simulink model "simulated_physical_reactor_v4_isolated"  (R2023a)
settings: Solver=FixedStepAuto  StartTime=0.0  StopTime=500  FixedStep=ts  RelTol=1e-3
values from neighbouring files (symbols this model uses):
  actionDelay = 10    [MainCode.m]
  buffer = 10    [MainCode.m]
  C0_attack_c = 0    [MainCode.m]
  C0_noise = 1    [MainCode.m]
  C0_post_attack = 0    [MainCode.m]
  C0_post_attack_val = -.25    (= -0.25)    [MainCode.m]
  Ccell0 = cell0 / v_cell    (= 15384.6153846)    [MainCode.m]
  CG0 = 185    [MainCode.m]
  CG_attack_c = 55    [MainCode.m]
  CG_attack_time = 175    [MainCode.m]
  CG_fake_failure = 0    [MainCode.m]
  CG_fake_failure_noise = 8    [MainCode.m]
  CG_increase_b = 0    [MainCode.m]
  CG_increase_rate = 2    [MainCode.m]
  cg_noGrowth = 10    [MainCode.m]
  CG_noise = 1    [MainCode.m]
  CG_post_attack = 1    [MainCode.m]
  CG_post_attack_val = .25    (= 0.25)    [MainCode.m]
  CG_ramp_attack = 1    [MainCode.m]
  CG_ramp_time = 125    [MainCode.m]
  CG_target = 50    [MainCode.m]
  CM = 4    [MainCode.m]
  CO0 = .245    (= 0.245)    [MainCode.m]
  CO_attack_time = 80    [MainCode.m]
  CO_fake_failure = 0    [MainCode.m]
  CO_fake_failure_mean = .08    (= 0.08)    [MainCode.m]
  CO_fake_failure_noise = .005    (= 0.005)    [MainCode.m]
  CO_ramp_attack = 0    [MainCode.m]
  CO_ramp_time = 100    [MainCode.m]
  count_thresh = 3    [MainCode.m]
  F_fresh_max = 25    [MainCode.m]
  F_net = F_fresh_start + F_recycle_start    (= 334.8)    [MainCode.m]
  flowrateNoiseActive = 0    [MainCode.m]
  flowrateNoiseVal = 0.5 / 100    (= 0.005)    [MainCode.m]
  fresh_attack = 0    [MainCode.m]
  fresh_attack_time = 70    [MainCode.m]
  fresh_attack_val = .1    (= 0.1)    [MainCode.m]
  freshPump_fail_time = 30    [MainCode.m]
  freshPump_failure = 0    [MainCode.m]
  freshPump_response_increases = 2    [MainCode.m]
  freshPump_response_window = 10    [MainCode.m]
  g_failure_start_t = 80    [MainCode.m]
  g_fault_wait_time = 10    [MainCode.m]
  g_flowrate_control_windowsize = 10    [MainCode.m]
  g_lownoise_val = 1.25    [MainCode.m]
  g_numpoints_fail = g_standdev_window_size+1    (= 16)    [MainCode.m]
  g_numpoints_low = 4    [MainCode.m]
  g_prob_arraylen = 15    [MainCode.m]
  g_prob_count = 6    [MainCode.m]
  g_prob_thresh = .45    (= 0.45)    [MainCode.m]
  g_standdev_window_size = 15    [MainCode.m]
  g_standev_tol = 7    [MainCode.m]
  glucose_fail_noise = 10    [MainCode.m]
  glucosesensor_failure = 0    [MainCode.m]
  lowConc_controller_onState = 1    [MainCode.m]
  mean_noise_C0 = 0    [MainCode.m]
  mean_noise_CG = 0    [MainCode.m]
  mu_max = 0.0251    [MainCode.m]
  n_size = t_window/ts    (= 2.5)    [MainCode.m]
  n_size_CG = n_size    (= 2.5)    [MainCode.m]
  o2_alpha = .20    (= 0.2)    [MainCode.m]
  o2_fail_mean = .008    (= 0.008)    [MainCode.m]
  o2_fail_noise = .005    (= 0.005)    [MainCode.m]
  o2_fail_time = 50    [MainCode.m]
  o2_fault_halfrange = .01    (= 0.01)    [MainCode.m]
  o2_fault_numpoints = 5    [MainCode.m]
  o2_lownoise_val = .0008    (= 0.0008)    [MainCode.m]
  o2_movingaverage_window = 10    [MainCode.m]
  o2_numpoints_low = 6    [MainCode.m]
  o2_prob_arraylen = 10    [MainCode.m]
  o2_prob_count = 6    [MainCode.m]
  o2_prob_thresh = .45    (= 0.45)    [MainCode.m]
  o2sensor_failure = 0    [MainCode.m]
  OCR = 2.8e-11    [MainCode.m]
  p_thresh = .4    (= 0.4)    [MainCode.m]
  rec_attack = 0    [MainCode.m]
  rec_attack_time = 50    [MainCode.m]
  rec_attack_val = 120    [MainCode.m]
  recPump_drop_val = .02    (= 0.02)    [MainCode.m]
  recPump_fail_time = 30    [MainCode.m]
  recPump_failure = 0    [MainCode.m]
  recPump_rollingavg_samples_buildup = 10    [MainCode.m]
  recPump_smallDrop_size = 0.006    [MainCode.m]
  stdev_noise_C0 = .002    (= 0.002)    [MainCode.m]
  stdev_noise_CG = 3.5    [MainCode.m]
  t_crit_CG = .7    (= 0.7)    [MainCode.m]
  ts = 1    [MainCode.m]
  V = 65.0    (= 65)    [MainCode.m]
  v_cell = 65    [MainCode.m]
  YGC = 155 * 10^-6    (= 0.000155)    [MainCode.m]
undefined symbols (not defined in the file or in its folder): DiscIntNeverNeededParam, recPump_numDrops_waitTime, recPump_rollingavg_numDrops
libraries: simulink x16, sldrtlib x11, dspstat3 x8, aerolibanimutils x1
(part 1 of 3)
settings Model: Creator=axtaw  LastModifiedBy=axtaw

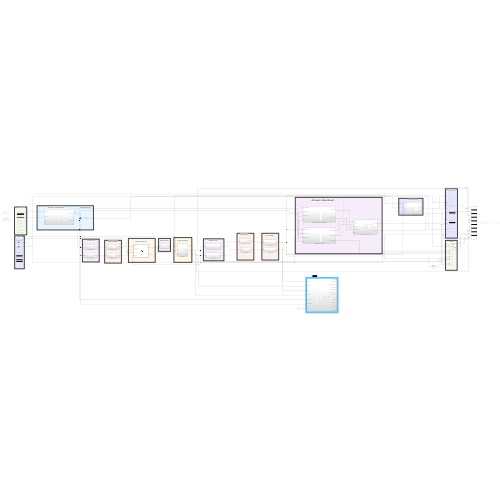
[thumbnail: Simulink's stored preview of the top-level diagram]
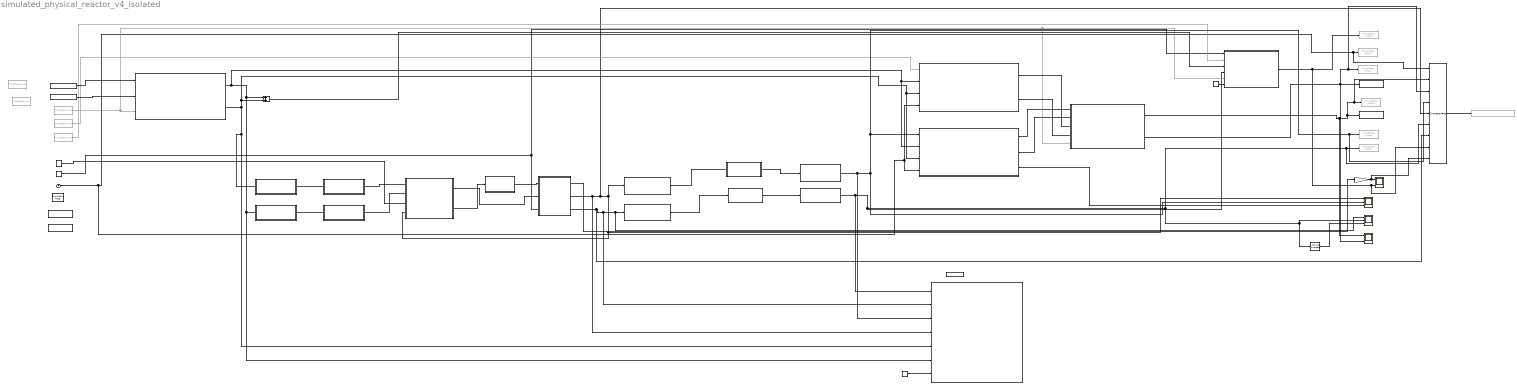
== system simulated_physical_reactor_v4_isolated ==
  note: Intended Flowrates
  note: Actuator Countermeasures
  note: Actuator Attacks
  note: Fluid Draw Selector
  note: Reactor Simulation
  note: Sensor Attacks
  note: Sensor Noise
  note: Scopes
  note: Constants
  note: System Inputs
  note: System Outputs
  note: Actuator Noise
  note: Actuator Faults
  note: Sensor Failure
  note: Actuator Adjustment
  note: Cell Count Estimatior
  Add : Sum
  Attack Response System : Subsystem
  Attack and Fault Detection System1 : Subsystem
  CG Attack System : Subsystem
  CG Sensor Noise System : Subsystem
  CO Attack System : Subsystem
  CO Sensor Noise System : Subsystem
  Cell Count : Scope  NumInputPorts=2
  Cell Count Estimation : sldrtlib/Internet of Things/ThingSpeak Output  Commented=on  DrvAddress=2409196  DrvOptions=[1 1 68 55 84 78 49 48 51 88 66 69 90 74 50 53 88 80 97 112 105 46 116 104 105 110 103 115 112 101 97 107 46 99 111 109 0 0 0 0 0 0 0 0 0 0 0 0 0 0 0 0 0 0 0 0 0 0 0 0 0 0 0 0 0 0 0 0 0 0 0 0 0 0 0 0 0 0 0 0 0 0 0 0 0 0 0 0 0 0 0 0 0 0 0 0 0 0 0 0 0 0 0 0 0 0 0 0 0 0 0 0 0 0 0 0 0 0 0 0 0 0 0 0 0 0 0 0 0 0 0 0 0 0 0 0 0 0 0 0 0 0 0 0 0 0 0 0 0 0 0 0 0 0 0 0 0 0 0 0 0 0 0 0 0 0 0 0 0 0 0 0 0 0 0 0 0 0 0 0 0 0 0 0 0 0 0 0 0 0 0 0 0 0 0 0 0 0 0 0 0 0 0 0 0 0 0 0 0 0 0 0 0 0 0 0 0 0 0 0 0 0 0 0 0 0 0 0 0 0 0 0 0 0 0 0 0 0 0 0 0 0 0 0 0 0 0 0 0 0 0 0 0 0 0 0]  SampleTime=ts  MaxMissedTicks=1000  ShowMissedTicks=off  YieldWhenWaiting=off  ChannelFields=4  OptParam=0  InitialValue=[]  FinalValue=[]
  Compromised Sensor Action System : Subsystem
  Constant : Constant  Value=ts
  Constant1 : Constant  Value=0
  DTR Fault Codes : sldrtlib/Internet of Things/ThingSpeak Input  Commented=on  DrvAddress=2409205  DrvOptions=[0 1 71 50 90 85 90 48 84 83 87 71 54 80 67 79 72 48 97 112 105 46 116 104 105 110 103 115 112 101 97 107 46 99 111 109 0 0 0 0 0 0 0 0 0 0 0 0 0 0 0 0 0 0 0 0 0 0 0 0 0 0 0 0 0 0 0 0 0 0 0 0 0 0 0 0 0 0 0 0 0 0 0 0 0 0 0 0 0 0 0 0 0 0 0 0 0 0 0 0 0 0 0 0 0 0 0 0 0 0 0 0 0 0 0 0 0 0 0 0 0 0 0 0 0 0 0 0 0 0 0 0 0 0 0 0 0 0 0 0 0 0 0 0 0 0 0 0 0 0 0 0 0 0 0 0 0 0 0 0 0 0 0 0 0 0 0 0 0 0 0 0 0 0 0 0 0 0 0 0 0 0 0 0 0 0 0 0 0 0 0 0 0 0 0 0 0 0 0 0 0 0 0 0 0 0 0 0 0 0 0 0 0 0 0 0 0 0 0 0 0 0 0 0 0 0 0 0 0 0 0 0 0 0 0 0 0 0 0 0 0 0 0 0 0 0 0 0 0 0 0 0 0 0 0 0]  SampleTime=ts  MaxMissedTicks=1000  ShowMissedTicks=off  YieldWhenWaiting=off  ChannelFields=3  OptParam=0  DataTypeStr=double
  DTR Glucose Concentration : sldrtlib/Internet of Things/ThingSpeak Input  Commented=on  DrvAddress=2409205  DrvOptions=[0 1 71 50 90 85 90 48 84 83 87 71 54 80 67 79 72 48 97 112 105 46 116 104 105 110 103 115 112 101 97 107 46 99 111 109 0 0 0 0 0 0 0 0 0 0 0 0 0 0 0 0 0 0 0 0 0 0 0 0 0 0 0 0 0 0 0 0 0 0 0 0 0 0 0 0 0 0 0 0 0 0 0 0 0 0 0 0 0 0 0 0 0 0 0 0 0 0 0 0 0 0 0 0 0 0 0 0 0 0 0 0 0 0 0 0 0 0 0 0 0 0 0 0 0 0 0 0 0 0 0 0 0 0 0 0 0 0 0 0 0 0 0 0 0 0 0 0 0 0 0 0 0 0 0 0 0 0 0 0 0 0 0 0 0 0 0 0 0 0 0 0 0 0 0 0 0 0 0 0 0 0 0 0 0 0 0 0 0 0 0 0 0 0 0 0 0 0 0 0 0 0 0 0 0 0 0 0 0 0 0 0 0 0 0 0 0 0 0 0 0 0 0 0 0 0 0 0 0 0 0 0 0 0 0 0 0 0 0 0 0 0 0 0 0 0 0 0 0 0 0 0 0 0 0 0]  SampleTime=ts  MaxMissedTicks=1000  ShowMissedTicks=off  YieldWhenWaiting=off  ChannelFields=4  OptParam=0  DataTypeStr=double
  DTR Oxygen Concentration : sldrtlib/Internet of Things/ThingSpeak Input  Commented=on  DrvAddress=2409205  DrvOptions=[0 1 71 50 90 85 90 48 84 83 87 71 54 80 67 79 72 48 97 112 105 46 116 104 105 110 103 115 112 101 97 107 46 99 111 109 0 0 0 0 0 0 0 0 0 0 0 0 0 0 0 0 0 0 0 0 0 0 0 0 0 0 0 0 0 0 0 0 0 0 0 0 0 0 0 0 0 0 0 0 0 0 0 0 0 0 0 0 0 0 0 0 0 0 0 0 0 0 0 0 0 0 0 0 0 0 0 0 0 0 0 0 0 0 0 0 0 0 0 0 0 0 0 0 0 0 0 0 0 0 0 0 0 0 0 0 0 0 0 0 0 0 0 0 0 0 0 0 0 0 0 0 0 0 0 0 0 0 0 0 0 0 0 0 0 0 0 0 0 0 0 0 0 0 0 0 0 0 0 0 0 0 0 0 0 0 0 0 0 0 0 0 0 0 0 0 0 0 0 0 0 0 0 0 0 0 0 0 0 0 0 0 0 0 0 0 0 0 0 0 0 0 0 0 0 0 0 0 0 0 0 0 0 0 0 0 0 0 0 0 0 0 0 0 0 0 0 0 0 0 0 0 0 0 0 0]  SampleTime=ts  MaxMissedTicks=1000  ShowMissedTicks=off  YieldWhenWaiting=off  ChannelFields=5  OptParam=0  DataTypeStr=double
  Data Store Memory : DataStoreMemory  DataStoreName=recycle_medium_flowrate  WriteAfterWriteMsg=warning  InitialValue=F_recycle_start  ShowAdditionalParam=off
  Data Store Memory1 : DataStoreMemory  DataStoreName=fresh_medium_flowrate  WriteAfterWriteMsg=warning  InitialValue=F_fresh_start  ShowAdditionalParam=off
  Data Store Memory2 : DataStoreMemory  DataStoreName=aliveTime  WriteAfterWriteMsg=warning  ShowAdditionalParam=off
  Data Store Read : DataStoreRead  DataStoreName=fresh_medium_flowrate  IndexOptions=Index vector (dialog)  Indices=1  OutputSizes=1
  Data Store Read1 : DataStoreRead  DataStoreName=recycle_medium_flowrate  IndexOptions=Index vector (dialog)  Indices=1  OutputSizes=1
  Data Store Write : DataStoreWrite  DataStoreName=fresh_medium_flowrate  IndexOptions=Index vector (dialog)  Indices=1  OutputSizes=1
  Data Store Write1 : DataStoreWrite  DataStoreName=recycle_medium_flowrate  IndexOptions=Index vector (dialog)  Indices=1  OutputSizes=1
  Flowrate Inconsistency System : Subsystem
  Flowrates : Scope  NumInputPorts=2
  Fresh Flowrate Attack System : Subsystem
  Fresh Flowrate Chosen : sldrtlib/Internet of Things/ThingSpeak Output  Commented=on  DrvAddress=2409196  DrvOptions=[1 1 68 55 84 78 49 48 51 88 66 69 90 74 50 53 88 80 97 112 105 46 116 104 105 110 103 115 112 101 97 107 46 99 111 109 0 0 0 0 0 0 0 0 0 0 0 0 0 0 0 0 0 0 0 0 0 0 0 0 0 0 0 0 0 0 0 0 0 0 0 0 0 0 0 0 0 0 0 0 0 0 0 0 0 0 0 0 0 0 0 0 0 0 0 0 0 0 0 0 0 0 0 0 0 0 0 0 0 0 0 0 0 0 0 0 0 0 0 0 0 0 0 0 0 0 0 0 0 0 0 0 0 0 0 0 0 0 0 0 0 0 0 0 0 0 0 0 0 0 0 0 0 0 0 0 0 0 0 0 0 0 0 0 0 0 0 0 0 0 0 0 0 0 0 0 0 0 0 0 0 0 0 0 0 0 0 0 0 0 0 0 0 0 0 0 0 0 0 0 0 0 0 0 0 0 0 0 0 0 0 0 0 0 0 0 0 0 0 0 0 0 0 0 0 0 0 0 0 0 0 0 0 0 0 0 0 0 0 0 0 0 0 0 0 0 0 0 0 0 0 0 0 0 0 0]  SampleTime=ts  MaxMissedTicks=1000  ShowMissedTicks=off  YieldWhenWaiting=off  ChannelFields=3  OptParam=0  InitialValue=[]  FinalValue=[]
  Fresh Flowrate Fault System : Subsystem
  Fresh Medium Flowrate Command : sldrtlib/Internet of Things/ThingSpeak Input  Commented=on  DrvAddress=2409205  DrvOptions=[0 1 71 50 90 85 90 48 84 83 87 71 54 80 67 79 72 48 97 112 105 46 116 104 105 110 103 115 112 101 97 107 46 99 111 109 0 0 0 0 0 0 0 0 0 0 0 0 0 0 0 0 0 0 0 0 0 0 0 0 0 0 0 0 0 0 0 0 0 0 0 0 0 0 0 0 0 0 0 0 0 0 0 0 0 0 0 0 0 0 0 0 0 0 0 0 0 0 0 0 0 0 0 0 0 0 0 0 0 0 0 0 0 0 0 0 0 0 0 0 0 0 0 0 0 0 0 0 0 0 0 0 0 0 0 0 0 0 0 0 0 0 0 0 0 0 0 0 0 0 0 0 0 0 0 0 0 0 0 0 0 0 0 0 0 0 0 0 0 0 0 0 0 0 0 0 0 0 0 0 0 0 0 0 0 0 0 0 0 0 0 0 0 0 0 0 0 0 0 0 0 0 0 0 0 0 0 0 0 0 0 0 0 0 0 0 0 0 0 0 0 0 0 0 0 0 0 0 0 0 0 0 0 0 0 0 0 0 0 0 0 0 0 0 0 0 0 0 0 0 0 0 0 0 0 0]  SampleTime=ts  MaxMissedTicks=1000  ShowMissedTicks=off  YieldWhenWaiting=off  ChannelFields=1  OptParam=0  DataTypeStr=double
  Fresh glucose concentration : Constant  Value=CG0
  Fresh oxygen concentration : Constant  Value=CO0
  Gain : Gain  Gain=v_cell
  Glucose Concentration Output : sldrtlib/Internet of Things/ThingSpeak Output  Commented=on  DrvAddress=2409196  DrvOptions=[1 1 68 55 84 78 49 48 51 88 66 69 90 74 50 53 88 80 97 112 105 46 116 104 105 110 103 115 112 101 97 107 46 99 111 109 0 0 0 0 0 0 0 0 0 0 0 0 0 0 0 0 0 0 0 0 0 0 0 0 0 0 0 0 0 0 0 0 0 0 0 0 0 0 0 0 0 0 0 0 0 0 0 0 0 0 0 0 0 0 0 0 0 0 0 0 0 0 0 0 0 0 0 0 0 0 0 0 0 0 0 0 0 0 0 0 0 0 0 0 0 0 0 0 0 0 0 0 0 0 0 0 0 0 0 0 0 0 0 0 0 0 0 0 0 0 0 0 0 0 0 0 0 0 0 0 0 0 0 0 0 0 0 0 0 0 0 0 0 0 0 0 0 0 0 0 0 0 0 0 0 0 0 0 0 0 0 0 0 0 0 0 0 0 0 0 0 0 0 0 0 0 0 0 0 0 0 0 0 0 0 0 0 0 0 0 0 0 0 0 0 0 0 0 0 0 0 0 0 0 0 0 0 0 0 0 0 0 0 0 0 0 0 0 0 0 0 0 0 0 0 0 0 0 0 0]  SampleTime=ts  MaxMissedTicks=1000  ShowMissedTicks=off  YieldWhenWaiting=off  ChannelFields=5  OptParam=0  InitialValue=[]  FinalValue=[]
  Glucose Concentrations : Scope  NumInputPorts=3
  Glucose sensor failure : Subsystem
  Moving Average : dspstat3/Moving Average  Method=Sliding window  ForgettingFactorPort=off  SpecifyWindowLength=on  WindowLength=4  OverlapLength=3  AllowArbitraryInputLength=off  ForgettingFactor=0.9  SimulateUsing=Code generation
  Oxygen Concentration Output : sldrtlib/Internet of Things/ThingSpeak Output  Commented=on  DrvAddress=2409196  DrvOptions=[1 1 68 55 84 78 49 48 51 88 66 69 90 74 50 53 88 80 97 112 105 46 116 104 105 110 103 115 112 101 97 107 46 99 111 109 0 0 0 0 0 0 0 0 0 0 0 0 0 0 0 0 0 0 0 0 0 0 0 0 0 0 0 0 0 0 0 0 0 0 0 0 0 0 0 0 0 0 0 0 0 0 0 0 0 0 0 0 0 0 0 0 0 0 0 0 0 0 0 0 0 0 0 0 0 0 0 0 0 0 0 0 0 0 0 0 0 0 0 0 0 0 0 0 0 0 0 0 0 0 0 0 0 0 0 0 0 0 0 0 0 0 0 0 0 0 0 0 0 0 0 0 0 0 0 0 0 0 0 0 0 0 0 0 0 0 0 0 0 0 0 0 0 0 0 0 0 0 0 0 0 0 0 0 0 0 0 0 0 0 0 0 0 0 0 0 0 0 0 0 0 0 0 0 0 0 0 0 0 0 0 0 0 0 0 0 0 0 0 0 0 0 0 0 0 0 0 0 0 0 0 0 0 0 0 0 0 0 0 0 0 0 0 0 0 0 0 0 0 0 0 0 0 0 0 0]  SampleTime=ts  MaxMissedTicks=1000  ShowMissedTicks=off  YieldWhenWaiting=off  ChannelFields=6  OptParam=0  InitialValue=[]  FinalValue=[]
  Oxygen Concentrations : Scope  NumInputPorts=3
  Oxygen sensor failure : Subsystem
  Reactor Clock : Clock
  Reactor Time : sldrtlib/Internet of Things/ThingSpeak Output  Commented=on  DrvAddress=2409196  DrvOptions=[1 1 68 55 84 78 49 48 51 88 66 69 90 74 50 53 88 80 97 112 105 46 116 104 105 110 103 115 112 101 97 107 46 99 111 109 0 0 0 0 0 0 0 0 0 0 0 0 0 0 0 0 0 0 0 0 0 0 0 0 0 0 0 0 0 0 0 0 0 0 0 0 0 0 0 0 0 0 0 0 0 0 0 0 0 0 0 0 0 0 0 0 0 0 0 0 0 0 0 0 0 0 0 0 0 0 0 0 0 0 0 0 0 0 0 0 0 0 0 0 0 0 0 0 0 0 0 0 0 0 0 0 0 0 0 0 0 0 0 0 0 0 0 0 0 0 0 0 0 0 0 0 0 0 0 0 0 0 0 0 0 0 0 0 0 0 0 0 0 0 0 0 0 0 0 0 0 0 0 0 0 0 0 0 0 0 0 0 0 0 0 0 0 0 0 0 0 0 0 0 0 0 0 0 0 0 0 0 0 0 0 0 0 0 0 0 0 0 0 0 0 0 0 0 0 0 0 0 0 0 0 0 0 0 0 0 0 0 0 0 0 0 0 0 0 0 0 0 0 0 0 0 0 0 0 0]  SampleTime=ts  MaxMissedTicks=1000  ShowMissedTicks=off  YieldWhenWaiting=off  ChannelFields=1  OptParam=0  InitialValue=[]  FinalValue=[]
  Recycle Flowrate Attack System : Subsystem
  Recycle Flowrate Chosen : sldrtlib/Internet of Things/ThingSpeak Output  Commented=on  DrvAddress=2409196  DrvOptions=[1 1 68 55 84 78 49 48 51 88 66 69 90 74 50 53 88 80 97 112 105 46 116 104 105 110 103 115 112 101 97 107 46 99 111 109 0 0 0 0 0 0 0 0 0 0 0 0 0 0 0 0 0 0 0 0 0 0 0 0 0 0 0 0 0 0 0 0 0 0 0 0 0 0 0 0 0 0 0 0 0 0 0 0 0 0 0 0 0 0 0 0 0 0 0 0 0 0 0 0 0 0 0 0 0 0 0 0 0 0 0 0 0 0 0 0 0 0 0 0 0 0 0 0 0 0 0 0 0 0 0 0 0 0 0 0 0 0 0 0 0 0 0 0 0 0 0 0 0 0 0 0 0 0 0 0 0 0 0 0 0 0 0 0 0 0 0 0 0 0 0 0 0 0 0 0 0 0 0 0 0 0 0 0 0 0 0 0 0 0 0 0 0 0 0 0 0 0 0 0 0 0 0 0 0 0 0 0 0 0 0 0 0 0 0 0 0 0 0 0 0 0 0 0 0 0 0 0 0 0 0 0 0 0 0 0 0 0 0 0 0 0 0 0 0 0 0 0 0 0 0 0 0 0 0 0]  SampleTime=ts  MaxMissedTicks=1000  ShowMissedTicks=off  YieldWhenWaiting=off  ChannelFields=2  OptParam=0  InitialValue=[]  FinalValue=[]
  Recycle Flowrate Fault System : Subsystem
  Recycle Medium Flowrate Command : sldrtlib/Internet of Things/ThingSpeak Input  Commented=on  DrvAddress=2409205  DrvOptions=[0 1 71 50 90 85 90 48 84 83 87 71 54 80 67 79 72 48 97 112 105 46 116 104 105 110 103 115 112 101 97 107 46 99 111 109 0 0 0 0 0 0 0 0 0 0 0 0 0 0 0 0 0 0 0 0 0 0 0 0 0 0 0 0 0 0 0 0 0 0 0 0 0 0 0 0 0 0 0 0 0 0 0 0 0 0 0 0 0 0 0 0 0 0 0 0 0 0 0 0 0 0 0 0 0 0 0 0 0 0 0 0 0 0 0 0 0 0 0 0 0 0 0 0 0 0 0 0 0 0 0 0 0 0 0 0 0 0 0 0 0 0 0 0 0 0 0 0 0 0 0 0 0 0 0 0 0 0 0 0 0 0 0 0 0 0 0 0 0 0 0 0 0 0 0 0 0 0 0 0 0 0 0 0 0 0 0 0 0 0 0 0 0 0 0 0 0 0 0 0 0 0 0 0 0 0 0 0 0 0 0 0 0 0 0 0 0 0 0 0 0 0 0 0 0 0 0 0 0 0 0 0 0 0 0 0 0 0 0 0 0 0 0 0 0 0 0 0 0 0 0 0 0 0 0 0]  SampleTime=ts  MaxMissedTicks=1000  ShowMissedTicks=off  YieldWhenWaiting=off  ChannelFields=2  OptParam=0  DataTypeStr=double
  Regular Process Control Adjustment : Subsystem
  Simulated Reactor : Subsystem
  Simulation Failsafe Process Control Adjustment1 : Subsystem
  Simulation Pace : aerolibanimutils/Simulation Pace  SimulationPace=500  SleepMode=Auto  OutputPaceError=off  SampleTime=ts
  Subsystem2 : Subsystem
  To File : ToFile  Commented=on  Filename=SPR_basicControl_run2.mat  SampleTime=ts
  Vector Concatenate : Concatenate  NumInputs=9
  recycle or fresh medium1 : MATLAB Function  TreatAsAtomicUnit=on
  wires:
  recycle or fresh medium1/1(CG_inlet) -> Simulated Reactor/2(CG0)
  Simulated Reactor/1(CCell) -> Gain/1
  CG Sensor Noise System/1(CG_out) -> Glucose sensor failure/1(In1)
  CO Sensor Noise System/1(CO_out) -> Oxygen sensor failure/1(CO_out)
  CO Attack System/1(CO_out) -> Attack and Fault Detection System1/1(CO_sensor), Subsystem2/4(exit_o2_actual), Vector Concatenate/6, Oxygen Concentration Output/1, Moving Average/1, Oxygen Concentrations/2  "oxygen sensor value"
  Reactor Clock/1 -> Vector Concatenate/1, Reactor Time/1, Simulation Failsafe Process Control Adjustment1/4(Time), Regular Process Control Adjustment/4(Time)  "reactor time"
  Fresh oxygen concentration/1 -> Subsystem2/1(Inlet_o2), Simulated Reactor/3(CO0)
  recycle or fresh medium1/2(total_flowrate) -> Flowrate Inconsistency System/1(input_flowrate)
  Attack Response System/2(Fresh Flowrate Out) -> Attack and Fault Detection System1/5(freshPump_flowrate), Fresh Flowrate Fault System/1(output_flowrate), Add/2, Simulation Failsafe Process Control Adjustment1/3(Old Fresh FLowrate), Regular Process Control Adjustment/3(Old Fresh FLowrate)  "fresh"
  Attack Response System/1(Recycle Flowrate Out) -> Add/1, Attack and Fault Detection System1/6(recyclePump_flowrate), Recycle Flowrate Fault System/1(output_flowrate), Simulation Failsafe Process Control Adjustment1/2(Old Recycle Flowrate), Regular Process Control Adjustment/2(Old Recycle Flowrate)  "recycle"
  Fresh glucose concentration/1 -> recycle or fresh medium1/3(CG0)
  Simulated Reactor/3(CO_outlet) -> Vector Concatenate/7, Attack and Fault Detection System1/2(CO_predicted), Oxygen Concentrations/1, CO Sensor Noise System/1(CO_in)  "actual oxygen value"
  Glucose sensor failure/1(Sensor g value) -> CG Attack System/1(CG_in)
  Oxygen sensor failure/1(CO_in) -> CO Attack System/1(CO_in)
  Simulated Reactor/2(CG_outlet) -> Attack and Fault Detection System1/4(CG_predicted1), Vector Concatenate/5, recycle or fresh medium1/4(CG_recycled), Glucose Concentrations/1, CG Sensor Noise System/1(CG_in)  "actual glucose value"
  Flowrate Inconsistency System/1(output_flowrate) -> Simulated Reactor/1(F)
  Regular Process Control Adjustment/1(New Fresh Flowrate) -> Compromised Sensor Action System/1(Actual_fresh)
  Regular Process Control Adjustment/2(New Recycle Flowrate) -> Compromised Sensor Action System/2(Actual_recycle)
  DTR Fault Codes/1 -> Attack Response System/3(Fault Code), Compromised Sensor Action System/5(faultCode), Subsystem2/5(faultCode)
  DTR Oxygen Concentration/1 -> Subsystem2/2(exit_o2_sim)
  Constant/1 -> Subsystem2/6(dt)
  Subsystem2/1(Cell count) -> Vector Concatenate/8, Cell Count/2, Cell Count Estimation/1  "estimated cell count"
  DTR Glucose Concentration/1 -> Simulation Failsafe Process Control Adjustment1/1(Glucose Concentration)
  Add/1 -> Subsystem2/3(net_flowrate)
  Data Store Read1/1 -> Attack Response System/1(Recycle Flowrate)
  Data Store Read/1 -> Attack Response System/2(Fresh Flowrate)
  Fresh Flowrate Fault System/1(Fresh Flowrate) -> Fresh Flowrate Attack System/1(flowrate_in)
  Recycle Flowrate Fault System/1(recycle Flowrate) -> Recycle Flowrate Attack System/1(flowrate_in)
  Recycle Flowrate Attack System/1(Recycle Flowrate) -> recycle or fresh medium1/2(recycled_flowrate)
  Fresh Flowrate Attack System/1(Fresh Flowrate) -> recycle or fresh medium1/1(fresh_flowrate)
  Compromised Sensor Action System/1(fresh_command) -> Flowrates/1, Vector Concatenate/2, Fresh Flowrate Chosen/1, Data Store Write/1  "fresh flowrate"
  Compromised Sensor Action System/2(recycle_command) -> Vector Concatenate/3, Recycle Flowrate Chosen/1, Flowrates/2, Data Store Write1/1  "recycle flowrate"
  Simulation Failsafe Process Control Adjustment1/2(New Recycle Flowrate) -> Compromised Sensor Action System/4(Simulated_recycle)
  Simulation Failsafe Process Control Adjustment1/1(New Fresh Flowrate) -> Compromised Sensor Action System/3(Simulated_fresh)
  CG Attack System/1(CG_out) -> Attack and Fault Detection System1/3(CG_sensor1), Regular Process Control Adjustment/1(Glucose Concentration), Vector Concatenate/4, Glucose Concentration Output/1, Glucose Concentrations/2  "glucose sensor value"
  Gain/1 -> Vector Concatenate/9, Cell Count/1  "actual cell count"
  Regular Process Control Adjustment/3(rolling average glucose) -> Glucose Concentrations/3
  Vector Concatenate/1 -> To File/1
  Moving Average/1 -> Oxygen Concentrations/3
  Constant1/1 -> Attack and Fault Detection System1/7(dnr)

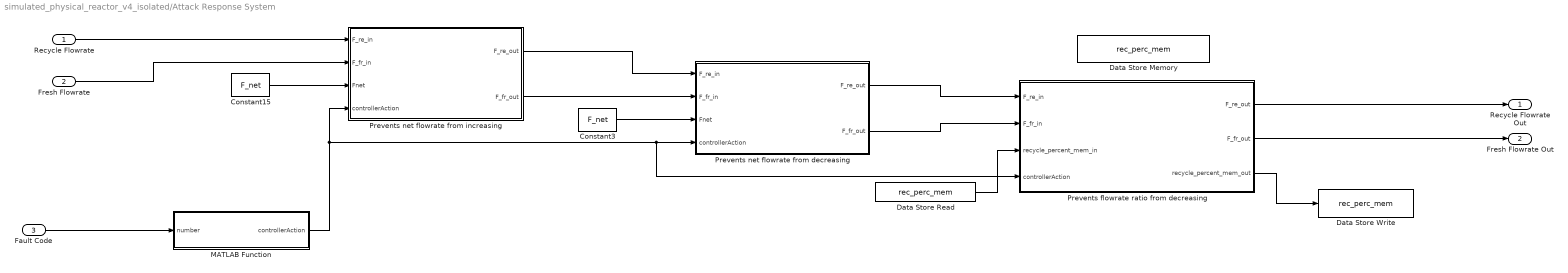
== system simulated_physical_reactor_v4_isolated/Attack Response System ==
  Recycle Flowrate : Inport
  Fresh Flowrate : Inport  Port=2
  Fault Code : Inport  Port=3
  Constant15 : Constant  Value=F_net
  Constant3 : Constant  Value=F_net
  Data Store Memory : DataStoreMemory  DataStoreName=rec_perc_mem  WriteAfterWriteMsg=warning  InitialValue=1  ShowAdditionalParam=off
  Data Store Read : DataStoreRead  DataStoreName=rec_perc_mem  IndexOptions=Index vector (dialog)  Indices=1  OutputSizes=1
  Data Store Write : DataStoreWrite  DataStoreName=rec_perc_mem  IndexOptions=Index vector (dialog)  Indices=1  OutputSizes=1
  MATLAB Function : MATLAB Function  TreatAsAtomicUnit=on
  Prevents flowrate ratio from decreasing : MATLAB Function  TreatAsAtomicUnit=on
  Prevents net flowrate from decreasing : MATLAB Function  TreatAsAtomicUnit=on
  Prevents net flowrate from increasing : MATLAB Function  TreatAsAtomicUnit=on
  Recycle Flowrate Out : Outport
  Fresh Flowrate Out : Outport  Port=2
  wires:
  Constant15/1 -> Prevents net flowrate from increasing/3(Fnet)
  MATLAB Function/1(controllerAction) -> Prevents flowrate ratio from decreasing/4(controllerAction), Prevents net flowrate from decreasing/4(controllerAction), Prevents net flowrate from increasing/4(controllerAction)
  Constant3/1 -> Prevents net flowrate from decreasing/3(Fnet)
  Prevents net flowrate from increasing/2(F_fr_out) -> Prevents net flowrate from decreasing/2(F_fr_in)
  Prevents net flowrate from increasing/1(F_re_out) -> Prevents net flowrate from decreasing/1(F_re_in)
  Data Store Read/1 -> Prevents flowrate ratio from decreasing/3(recycle_percent_mem_in)
  Prevents net flowrate from decreasing/1(F_re_out) -> Prevents flowrate ratio from decreasing/1(F_re_in)
  Prevents net flowrate from decreasing/2(F_fr_out) -> Prevents flowrate ratio from decreasing/2(F_fr_in)
  Prevents flowrate ratio from decreasing/3(recycle_percent_mem_out) -> Data Store Write/1
  Recycle Flowrate/1 -> Prevents net flowrate from increasing/1(F_re_in)
  Fresh Flowrate/1 -> Prevents net flowrate from increasing/2(F_fr_in)
  Prevents flowrate ratio from decreasing/1(F_re_out) -> Recycle Flowrate Out/1
  Prevents flowrate ratio from decreasing/2(F_fr_out) -> Fresh Flowrate Out/1
  Fault Code/1 -> MATLAB Function/1(number)

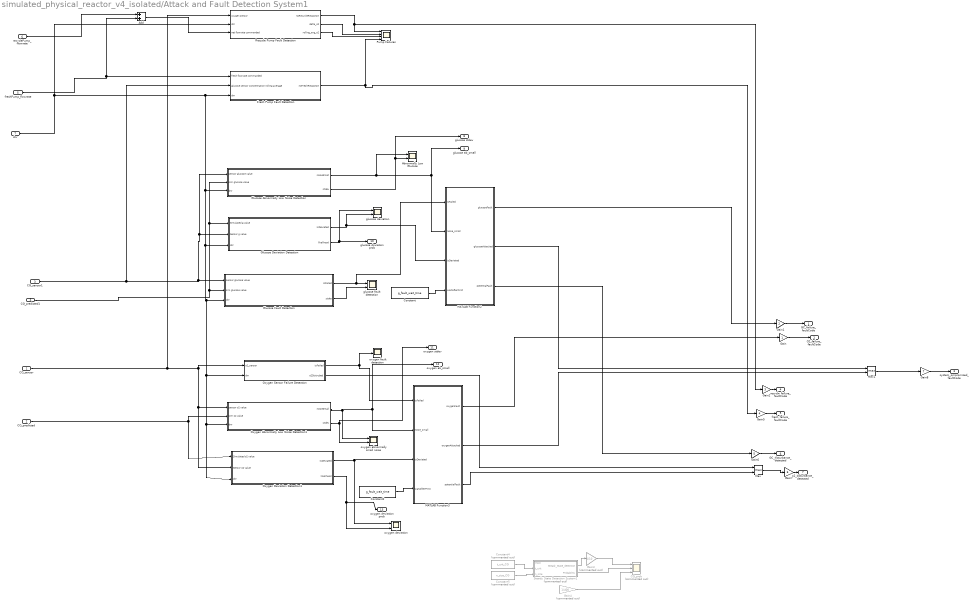
== system simulated_physical_reactor_v4_isolated/Attack and Fault Detection System1 ==
  CO_sensor : Inport
  CO_predicted : Inport  Port=2
  CG_sensor1 : Inport  Port=3
  CG_predicted1 : Inport  Port=4
  freshPump_flowrate : Inport  Port=5
  recyclePump_flowrate : Inport  Port=6
  dnr : Inport  Port=7
  Abnormally Low Glucose : Scope  NumInputPorts=2
  Add : Sum
  CG_prob : Scope  Commented=on  NumInputPorts=3
  Constant : Constant  Value=g_fault_wait_time
  Constant2 : Constant  Value=g_fault_wait_time
  Constant4 : Constant  Commented=on  Value=t_crit_CG
  Constant5 : Constant  Commented=on  Value=n_size_CG
  Fresh Pump Fault Detection : Subsystem
  Gain : Gain
  Gain1 : Gain  Gain=2
  Gain2 : Gain  Gain=3
  Gain3 : Gain  Commented=on  Gain=1/10
  Gain4 : Gain  Commented=on  Gain=1/400
  Gain5 : Gain  Gain=4
  Gain6 : Gain  Gain=5
  Gain7 : Gain  Gain=6
  Gain8 : Gain  Gain=7
  Glucose Abnormally Low Noise Detection : Subsystem
  Glucose Deviation Detection : Subsystem
  Glucose Fault Detection : Subsystem
  MATLAB Function2 : MATLAB Function  TreatAsAtomicUnit=on
  MATLAB Function3 : MATLAB Function  TreatAsAtomicUnit=on
  Max : MinMax  Function=max  Inputs=2
  Max1 : MinMax  Function=max  Inputs=2
  Oxygen Abnormally Low Noise Detection1 : Subsystem
  Oxygen Deviation Detection1 : Subsystem
  Oxygen Sensor Failure Detection : Subsystem
  Pump Failures : Scope  NumInputPorts=4
  Recycle Pump Fault Detection : Subsystem
  Steady State Detection System1 : Subsystem  Commented=on
  glucose deviation : Scope  NumInputPorts=2
  glucose fault detection : Scope  NumInputPorts=2
  oxygen abnormally small noise : Scope  NumInputPorts=2
  oxygen deviation : Scope  NumInputPorts=2
  oxygen fault detection : Scope
  GC_failure_faultCode : Outport
  O2_failure_faultCode : Outport  Port=2
  system_ompromised_faultCode : Outport  Port=3
  recycle_failure_faultCode : Outport  Port=4
  fresh_failure_faultCode : Outport  Port=5
  GC_disturbance_detected : Outport  Port=6
  o2_disturbance_detected : Outport  Port=7
  glucose stdev : Outport  Port=8
  glucose ab_small : Outport  Port=9
  glucose deviation prob : Outport  Port=10
  oxygen stdev : Outport  Port=11
  oxygen ab_small : Outport  Port=12
  oxygen deviation prob : Outport  Port=13
  wires:
  CO_sensor/1 -> Recycle Pump Fault Detection/1(oxygen sensor), Oxygen Deviation Detection1/2(Sensor o2 value), Oxygen Abnormally Low Noise Detection1/1(sensor o2 value), Oxygen Sensor Failure Detection/1(o2_sensor)
  CG_sensor1/1 -> Fresh Pump Fault Detection/2(glucose sensor concentration rolling average), Glucose Abnormally Low Noise Detection/1(sensor glucose value), Glucose Deviation Detection/2(Sensor g value), Glucose Fault Detection/1(sensor glucose value)
  CG_predicted1/1 -> Glucose Abnormally Low Noise Detection/2(sim glucose value), Glucose Deviation Detection/1(Simulated g value), Glucose Fault Detection/2(sim glucose value)
  Gain4/1 -> CG_prob/3
  Gain3/1 -> CG_prob/1
  Constant4/1 -> Steady State Detection System1/2(t_crit)
  Steady State Detection System1/1(Steady_State_detection) -> Gain3/1
  Constant5/1 -> Steady State Detection System1/3(n_size)
  Steady State Detection System1/2(Probability) -> CG_prob/2
  CO_predicted/1 -> Oxygen Deviation Detection1/1(Simulated o2 value), Oxygen Abnormally Low Noise Detection1/2(sim o2 value)
  Glucose Abnormally Low Noise Detection/1(noiseSmall) -> Abnormally Low Glucose/1, glucose ab_small/1, MATLAB Function2/2(noise_small)
  Glucose Deviation Detection/1(isDeviated) -> glucose deviation/2, MATLAB Function2/3(isDeviated)
  Glucose Fault Detection/1(isFailed) -> MATLAB Function2/1(isFailed), glucose fault detection/1
  Constant/1 -> MATLAB Function2/4(waitAfterFirst)
  MATLAB Function2/3(potentialFault) -> Gain6/1
  MATLAB Function2/2(glucoseAttacked) -> Max1/1
  MATLAB Function2/1(glucoseFault) -> Gain1/1
  Glucose Abnormally Low Noise Detection/2(stdev) -> glucose stdev/1, Abnormally Low Glucose/2
  Constant2/1 -> MATLAB Function3/4(waitAfterFirst)
  Oxygen Sensor Failure Detection/1(isFailed) -> oxygen fault detection/1, MATLAB Function3/1(isFailed)
  Oxygen Abnormally Low Noise Detection1/1(noiseSmall) -> MATLAB Function3/2(noise_small), oxygen ab_small/1, oxygen abnormally small noise/1
  Oxygen Deviation Detection1/1(isDeviated) -> MATLAB Function3/3(isDeviated), oxygen deviation/1
  Oxygen Abnormally Low Noise Detection1/2(stdev) -> oxygen stdev/1, oxygen abnormally small noise/2
  Oxygen Deviation Detection1/2(likelihood) -> oxygen deviation prob/1, oxygen deviation/2
  MATLAB Function3/3(potentialFault) -> Max/2
  MATLAB Function3/2(oxygenAttacked) -> Max1/2
  MATLAB Function3/1(oxygenFault) -> Gain/1
  freshPump_flowrate/1 -> Add/2, Fresh Pump Fault Detection/1(fresh flowrate commanded)
  Fresh Pump Fault Detection/1(noFreshResponse) -> Gain5/1, Pump Failures/4
  Glucose Deviation Detection/2(likelihood) -> glucose deviation prob/1, glucose deviation/1
  Glucose Fault Detection/2(stdev) -> glucose fault detection/2
  recyclePump_flowrate/1 -> Add/1
  Add/1 -> Recycle Pump Fault Detection/3(net flowrate commanded)
  Recycle Pump Fault Detection/1(noRecycleResponse) -> Pump Failures/1, Gain2/1
  Recycle Pump Fault Detection/2(delta_o2) -> Pump Failures/2
  Recycle Pump Fault Detection/3(rolling_avg_o2) -> Pump Failures/3
  Max1/1 -> Gain8/1
  Oxygen Sensor Failure Detection/2(o2Distrubed) -> Max/1
  Max/1 -> Gain7/1
  dnr/1 -> Oxygen Deviation Detection1/3(dnr), Oxygen Abnormally Low Noise Detection1/3(dnr), Oxygen Sensor Failure Detection/2(dnr), Glucose Fault Detection/3(dnr), Glucose Deviation Detection/3(dnr), Glucose Abnormally Low Noise Detection/3(dnr), Fresh Pump Fault Detection/3(dnr), Recycle Pump Fault Detection/2(dnr)
  Gain/1 -> O2_failure_faultCode/1
  Gain1/1 -> GC_failure_faultCode/1
  Gain2/1 -> recycle_failure_faultCode/1
  Gain5/1 -> fresh_failure_faultCode/1
  Gain6/1 -> GC_disturbance_detected/1
  Gain7/1 -> o2_disturbance_detected/1
  Gain8/1 -> system_ompromised_faultCode/1

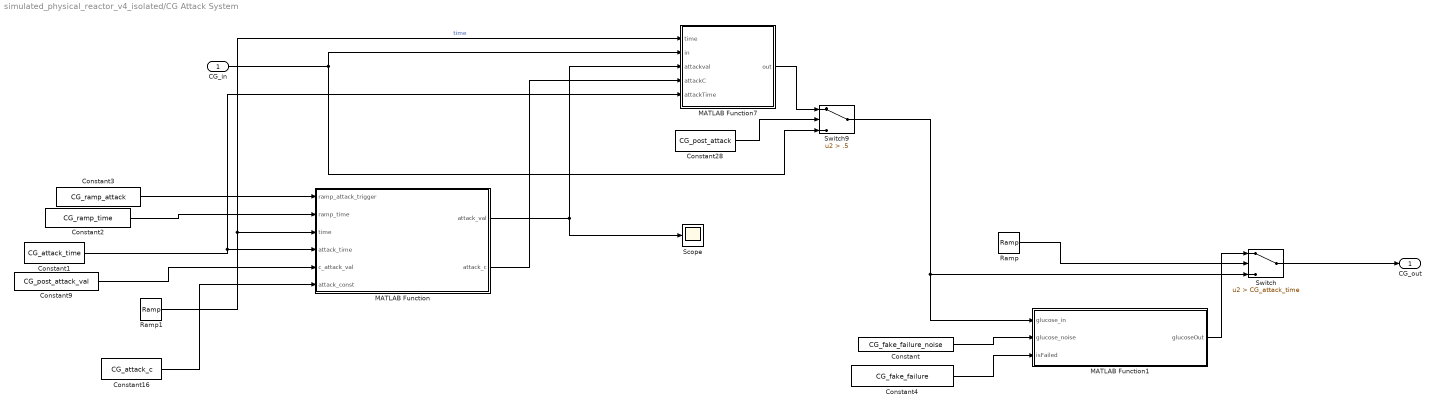
== system simulated_physical_reactor_v4_isolated/CG Attack System ==
  CG_in : Inport
  Constant : Constant  Value=CG_fake_failure_noise
  Constant1 : Constant  Value=CG_attack_time
  Constant16 : Constant  Value=CG_attack_c
  Constant2 : Constant  Value=CG_ramp_time
  Constant28 : Constant  Value=CG_post_attack
  Constant3 : Constant  Value=CG_ramp_attack
  Constant4 : Constant  Value=CG_fake_failure
  Constant9 : Constant  Value=CG_post_attack_val
  MATLAB Function : MATLAB Function  TreatAsAtomicUnit=on
  MATLAB Function1 : MATLAB Function  TreatAsAtomicUnit=on
  MATLAB Function7 : MATLAB Function  TreatAsAtomicUnit=on
  Ramp : simulink/Sources/Ramp  slope=1  start=0  InitialOutput=0
  Ramp1 : simulink/Sources/Ramp  slope=1  start=0  InitialOutput=0
  Scope : Scope
  Switch : Switch  Criteria=u2 > Threshold  Threshold=CG_attack_time  SaturateOnIntegerOverflow=off  InputSameDT=off
  Switch9 : Switch  Criteria=u2 > Threshold  Threshold=.5  SaturateOnIntegerOverflow=off  InputSameDT=off
  CG_out : Outport
  wires:
  Constant28/1 -> Switch9/2
  Ramp1/1 -> MATLAB Function/3(time), MATLAB Function7/1(time)  "time"
  MATLAB Function7/1(out) -> Switch9/1
  CG_in/1 -> Switch9/3, MATLAB Function7/2(in)
  Constant1/1 -> MATLAB Function7/5(attackTime), MATLAB Function/4(attack_time)
  Constant2/1 -> MATLAB Function/2(ramp_time)
  Constant3/1 -> MATLAB Function/1(ramp_attack_trigger)
  MATLAB Function/1(attack_val) -> Scope/1, MATLAB Function7/3(attackval)
  Constant9/1 -> MATLAB Function/5(c_attack_val)
  Constant/1 -> MATLAB Function1/2(glucose_noise)
  Ramp/1 -> Switch/2
  Switch9/1 -> MATLAB Function1/1(glucose_in), Switch/3
  MATLAB Function1/1(glucoseOut) -> Switch/1
  Constant4/1 -> MATLAB Function1/3(isFailed)
  Switch/1 -> CG_out/1
  MATLAB Function/2(attack_c) -> MATLAB Function7/4(attackC)
  Constant16/1 -> MATLAB Function/6(attack_const)

== system simulated_physical_reactor_v4_isolated/CG Sensor Noise System ==
  CG_in : Inport
  Constant24 : Constant  Value=mean_noise_CG
  Constant25 : Constant  Value=stdev_noise_CG
  Constant26 : Constant  Value=CG_noise
  MATLAB Function6 : MATLAB Function  TreatAsAtomicUnit=on
  Switch8 : Switch  Criteria=u2 > Threshold  SaturateOnIntegerOverflow=off  InputSameDT=off
  CG_out : Outport
  wires:
  Constant26/1 -> Switch8/2
  Constant25/1 -> MATLAB Function6/2(std)
  Constant24/1 -> MATLAB Function6/1(mean)
  MATLAB Function6/1(C_noisy) -> Switch8/1
  CG_in/1 -> Switch8/3, MATLAB Function6/3(C)
  Switch8/1 -> CG_out/1

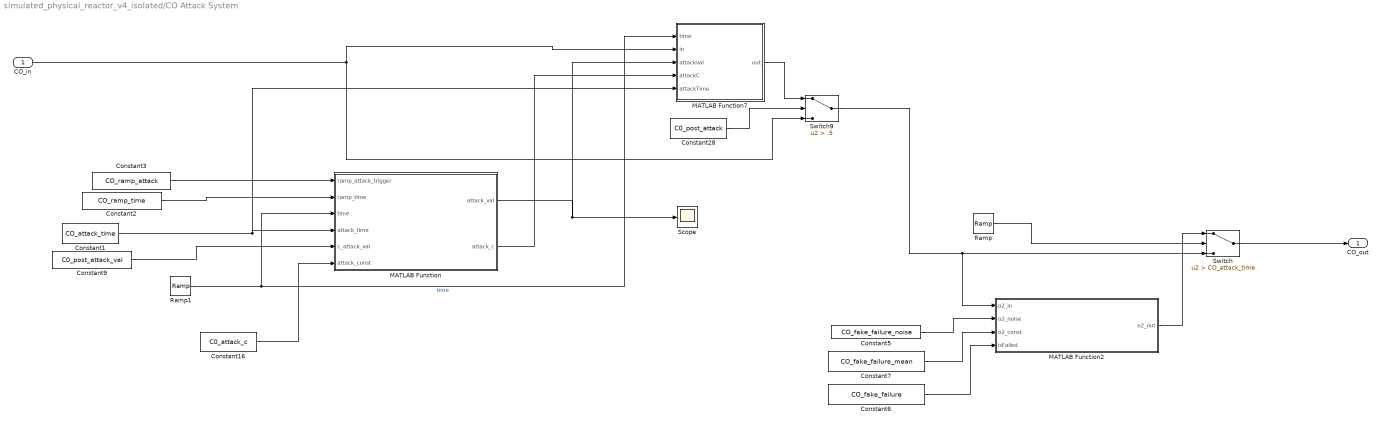
== system simulated_physical_reactor_v4_isolated/CO Attack System ==
  CO_in : Inport
  Constant1 : Constant  Value=CO_attack_time
  Constant16 : Constant  Value=C0_attack_c
  Constant2 : Constant  Value=CO_ramp_time
  Constant28 : Constant  Value=C0_post_attack
  Constant3 : Constant  Value=CO_ramp_attack
  Constant5 : Constant  Value=CO_fake_failure_noise
  Constant6 : Constant  Value=CO_fake_failure
  Constant7 : Constant  Value=CO_fake_failure_mean
  Constant9 : Constant  Value=C0_post_attack_val
  MATLAB Function : MATLAB Function  TreatAsAtomicUnit=on
  MATLAB Function2 : MATLAB Function  TreatAsAtomicUnit=on
  MATLAB Function7 : MATLAB Function  TreatAsAtomicUnit=on
  Ramp : simulink/Sources/Ramp  slope=1  start=0  InitialOutput=0
  Ramp1 : simulink/Sources/Ramp  slope=1  start=0  InitialOutput=0
  Scope : Scope
  Switch : Switch  Criteria=u2 > Threshold  Threshold=CO_attack_time  SaturateOnIntegerOverflow=off  InputSameDT=off
  Switch9 : Switch  Criteria=u2 > Threshold  Threshold=.5  SaturateOnIntegerOverflow=off  InputSameDT=off
  CO_out : Outport
  wires:
  MATLAB Function/1(attack_val) -> Scope/1, MATLAB Function7/3(attackval)
  Constant1/1 -> MATLAB Function7/5(attackTime), MATLAB Function/4(attack_time)
  Constant3/1 -> MATLAB Function/1(ramp_attack_trigger)
  Constant2/1 -> MATLAB Function/2(ramp_time)
  Switch/1 -> CO_out/1
  MATLAB Function7/1(out) -> Switch9/1
  Ramp1/1 -> MATLAB Function/3(time), MATLAB Function7/1(time)  "time"
  CO_in/1 -> MATLAB Function7/2(in), Switch9/3
  Constant28/1 -> Switch9/2
  Constant9/1 -> MATLAB Function/5(c_attack_val)
  Ramp/1 -> Switch/2
  Constant5/1 -> MATLAB Function2/2(o2_noise)
  Constant7/1 -> MATLAB Function2/3(o2_const)
  Switch9/1 -> MATLAB Function2/1(o2_in), Switch/3
  Constant6/1 -> MATLAB Function2/4(isFailed)
  MATLAB Function2/1(o2_out) -> Switch/1
  Constant16/1 -> MATLAB Function/6(attack_const)
  MATLAB Function/2(attack_c) -> MATLAB Function7/4(attackC)

== system simulated_physical_reactor_v4_isolated/CO Sensor Noise System ==
  CO_in : Inport
  Constant37 : Constant  Value=mean_noise_C0
  Constant38 : Constant  Value=stdev_noise_C0
  Constant39 : Constant  Value=C0_noise
  MATLAB Function14 : MATLAB Function  TreatAsAtomicUnit=on
  Switch15 : Switch  Criteria=u2 > Threshold  SaturateOnIntegerOverflow=off  InputSameDT=off
  CO_out : Outport
  wires:
  Constant37/1 -> MATLAB Function14/1(mean)
  MATLAB Function14/1(C_noisy) -> Switch15/1
  Constant38/1 -> MATLAB Function14/2(std)
  Constant39/1 -> Switch15/2
  CO_in/1 -> Switch15/3, MATLAB Function14/3(C)
  Switch15/1 -> CO_out/1

== system simulated_physical_reactor_v4_isolated/Compromised Sensor Action System ==
  Actual_fresh : Inport
  Actual_recycle : Inport  Port=2
  Simulated_fresh : Inport  Port=3
  Simulated_recycle : Inport  Port=4
  faultCode : Inport  Port=5
  MATLAB Function : MATLAB Function  TreatAsAtomicUnit=on
  MATLAB Function1 : MATLAB Function  TreatAsAtomicUnit=on
  fresh_command : Outport
  recycle_command : Outport  Port=2
  wires:
  Simulated_fresh/1 -> MATLAB Function/1(sim_fresh)
  Simulated_recycle/1 -> MATLAB Function/3(sim_rec)
  MATLAB Function1/1(ignoreSensor) -> MATLAB Function/5(ignoreSensor)
  Actual_fresh/1 -> fresh_command/1
  Actual_recycle/1 -> recycle_command/1
  faultCode/1 -> MATLAB Function1/1(number)

== system simulated_physical_reactor_v4_isolated/Flowrate Inconsistency System ==
  input_flowrate : Inport
  Constant : Constant  Value=flowrateNoiseVal
  Constant1 : Constant  Value=flowrateNoiseActive
  MATLAB Function : MATLAB Function  TreatAsAtomicUnit=on
  output_flowrate : Outport
  wires:
  input_flowrate/1 -> MATLAB Function/1(input_flowrate)
  MATLAB Function/1(output_flowrate) -> output_flowrate/1
  Constant/1 -> MATLAB Function/2(noise_percentage)
  Constant1/1 -> MATLAB Function/3(isActive)

== system simulated_physical_reactor_v4_isolated/Fresh Flowrate Attack System ==
  flowrate_in : Inport
  Constant : Constant  Value=fresh_attack
  Constant1 : Constant  Value=fresh_attack_val
  Constant2 : Constant  Value=fresh_attack_time
  MATLAB Function : MATLAB Function  TreatAsAtomicUnit=on
  Ramp : simulink/Sources/Ramp  slope=1  start=0  InitialOutput=0
  Fresh Flowrate : Outport
  wires:
  flowrate_in/1 -> MATLAB Function/1(flow_in)
  MATLAB Function/1(flow_out) -> Fresh Flowrate/1
  Constant/1 -> MATLAB Function/2(attack_on)
  Constant1/1 -> MATLAB Function/3(attack_val)
  Ramp/1 -> MATLAB Function/5(time)
  Constant2/1 -> MATLAB Function/4(attack_time)

== system simulated_physical_reactor_v4_isolated/Fresh Flowrate Fault System ==
  output_flowrate : Inport
  Constant : Constant  Value=freshPump_failure
  Constant1 : Constant  Value=freshPump_fail_time
  MATLAB Function : MATLAB Function  TreatAsAtomicUnit=on
  Ramp : simulink/Sources/Ramp  slope=1  start=0  InitialOutput=0
  Fresh Flowrate : Outport
  wires:
  output_flowrate/1 -> MATLAB Function/1(in_flow)
  MATLAB Function/1(out_flow) -> Fresh Flowrate/1
  Constant/1 -> MATLAB Function/2(fault_on)
  Constant1/1 -> MATLAB Function/4(fault_time)
  Ramp/1 -> MATLAB Function/3(time)

== system simulated_physical_reactor_v4_isolated/Glucose sensor failure ==
  In1 : Inport
  Constant : Constant  Value=glucose_fail_noise
  Constant1 : Constant  Value=glucosesensor_failure
  MATLAB Function : MATLAB Function  TreatAsAtomicUnit=on
  Ramp : simulink/Sources/Ramp  slope=1  start=0  InitialOutput=0
  Switch : Switch  Criteria=u2 > Threshold  Threshold=g_failure_start_t  SaturateOnIntegerOverflow=off  InputSameDT=off
  Sensor g value : Outport
  wires:
  In1/1 -> MATLAB Function/1(glucose_in), Switch/3
  MATLAB Function/1(glucoseOut) -> Switch/1
  Constant1/1 -> MATLAB Function/3(isFailed)
  Constant/1 -> MATLAB Function/2(glucose_noise)
  Ramp/1 -> Switch/2
  Switch/1 -> Sensor g value/1

== system simulated_physical_reactor_v4_isolated/Oxygen sensor failure ==
  CO_out : Inport
  Constant : Constant  Value=o2_fail_noise
  Constant1 : Constant  Value=o2sensor_failure
  Constant2 : Constant  Value=o2_fail_mean
  Constant3 : Constant  Value=o2_fail_time
  MATLAB Function : MATLAB Function  TreatAsAtomicUnit=on
  Ramp : simulink/Sources/Ramp  slope=1  start=0  InitialOutput=0
  CO_in : Outport
  wires:
  Constant1/1 -> MATLAB Function/4(isFailed)
  MATLAB Function/1(o2_out) -> CO_in/1
  CO_out/1 -> MATLAB Function/1(o2_in)
  Constant/1 -> MATLAB Function/2(o2_noise)
  Constant2/1 -> MATLAB Function/3(o2_const)
  Ramp/1 -> MATLAB Function/6(time)
  Constant3/1 -> MATLAB Function/5(o2_fail_time)

== system simulated_physical_reactor_v4_isolated/Recycle Flowrate Attack System ==
  flowrate_in : Inport
  Constant : Constant  Value=rec_attack
  Constant1 : Constant  Value=rec_attack_val
  Constant2 : Constant  Value=rec_attack_time
  MATLAB Function : MATLAB Function  TreatAsAtomicUnit=on
  Ramp : simulink/Sources/Ramp  slope=1  start=0  InitialOutput=0
  Recycle Flowrate : Outport
  wires:
  Constant2/1 -> MATLAB Function/4(attack_time)
  Ramp/1 -> MATLAB Function/5(time)
  Constant1/1 -> MATLAB Function/3(attack_val)
  Constant/1 -> MATLAB Function/2(attack_on)
  MATLAB Function/1(flow_out) -> Recycle Flowrate/1
  flowrate_in/1 -> MATLAB Function/1(flow_in)

== system simulated_physical_reactor_v4_isolated/Recycle Flowrate Fault System ==
  output_flowrate : Inport
  Constant : Constant  Value=recPump_failure
  Constant1 : Constant  Value=recPump_fail_time
  MATLAB Function : MATLAB Function  TreatAsAtomicUnit=on
  Ramp : simulink/Sources/Ramp  slope=1  start=0  InitialOutput=0
  recycle Flowrate : Outport
  wires:
  output_flowrate/1 -> MATLAB Function/1(in_flow)
  MATLAB Function/1(out_flow) -> recycle Flowrate/1
  Constant/1 -> MATLAB Function/2(fault_on)
  Constant1/1 -> MATLAB Function/4(fault_time)
  Ramp/1 -> MATLAB Function/3(time)

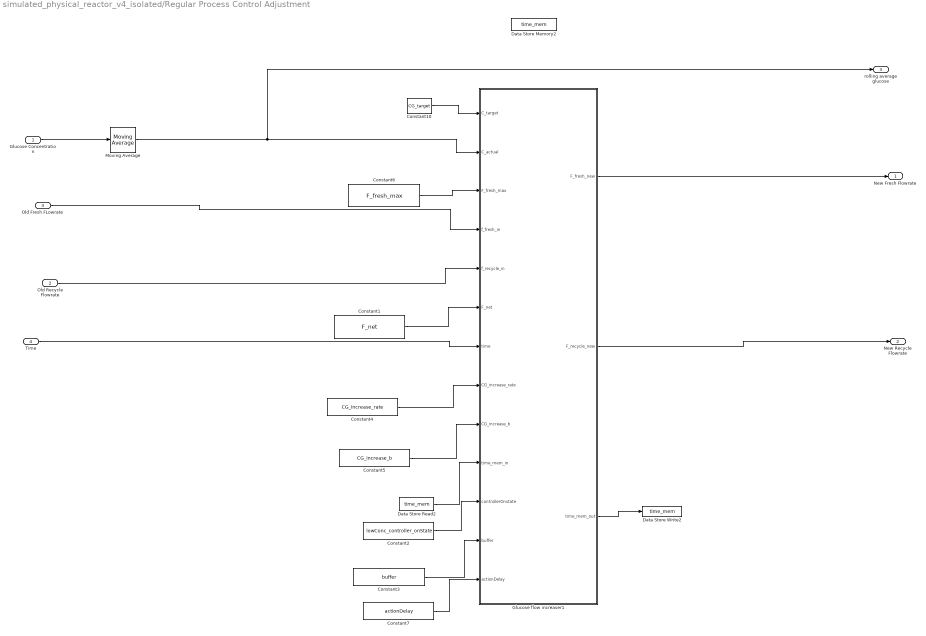
== system simulated_physical_reactor_v4_isolated/Regular Process Control Adjustment ==
  Glucose Concentration : Inport
  Old Recycle Flowrate : Inport  Port=2
  Old Fresh FLowrate : Inport  Port=3
  Time : Inport  Port=4
  Constant1 : Constant  Value=F_net
  Constant10 : Constant  Value=CG_target
  Constant2 : Constant  Value=lowConc_controller_onState
  Constant3 : Constant  Value=buffer
  Constant4 : Constant  Value=CG_increase_rate
  Constant5 : Constant  Value=CG_increase_b
  Constant6 : Constant  Value=F_fresh_max
  Constant7 : Constant  Value=actionDelay
  Data Store Memory2 : DataStoreMemory  DataStoreName=time_mem  WriteAfterWriteMsg=warning  ShowAdditionalParam=off
  Data Store Read2 : DataStoreRead  DataStoreName=time_mem  IndexOptions=Index vector (dialog)  Indices=1  OutputSizes=1
  Data Store Write2 : DataStoreWrite  DataStoreName=time_mem  IndexOptions=Index vector (dialog)  Indices=1  OutputSizes=1
  Glucose flow increaser1 : MATLAB Function  TreatAsAtomicUnit=on
  Moving Average : dspstat3/Moving Average  Method=Sliding window  ForgettingFactorPort=off  SpecifyWindowLength=on  WindowLength=g_flowrate_control_windowsize  OverlapLength=g_flowrate_control_windowsize-1  AllowArbitraryInputLength=off  ForgettingFactor=0.9  SimulateUsing=Code generation
  New Fresh Flowrate : Outport
  New Recycle Flowrate : Outport  Port=2
  rolling average glucose : Outport  Port=3
  wires:
  Time/1 -> Glucose flow increaser1/7(time)
  Constant10/1 -> Glucose flow increaser1/1(C_target)
  Glucose Concentration/1 -> Moving Average/1
  Constant4/1 -> Glucose flow increaser1/8(CG_increase_rate)
  Glucose flow increaser1/3(time_mem_out) -> Data Store Write2/1
  Data Store Read2/1 -> Glucose flow increaser1/10(time_mem_in)
  Constant5/1 -> Glucose flow increaser1/9(CG_increase_b)
  Constant6/1 -> Glucose flow increaser1/3(F_fresh_max)
  Constant2/1 -> Glucose flow increaser1/11(controllerOnstate)
  Constant3/1 -> Glucose flow increaser1/12(buffer)
  Constant1/1 -> Glucose flow increaser1/6(F_net)
  Old Recycle Flowrate/1 -> Glucose flow increaser1/5(f_recycle_in)
  Old Fresh FLowrate/1 -> Glucose flow increaser1/4(f_fresh_in)
  Glucose flow increaser1/1(F_fresh_new) -> New Fresh Flowrate/1
  Glucose flow increaser1/2(F_recycle_new) -> New Recycle Flowrate/1
  Moving Average/1 -> rolling average glucose/1, Glucose flow increaser1/2(C_actual)
  Constant7/1 -> Glucose flow increaser1/13(actionDelay)

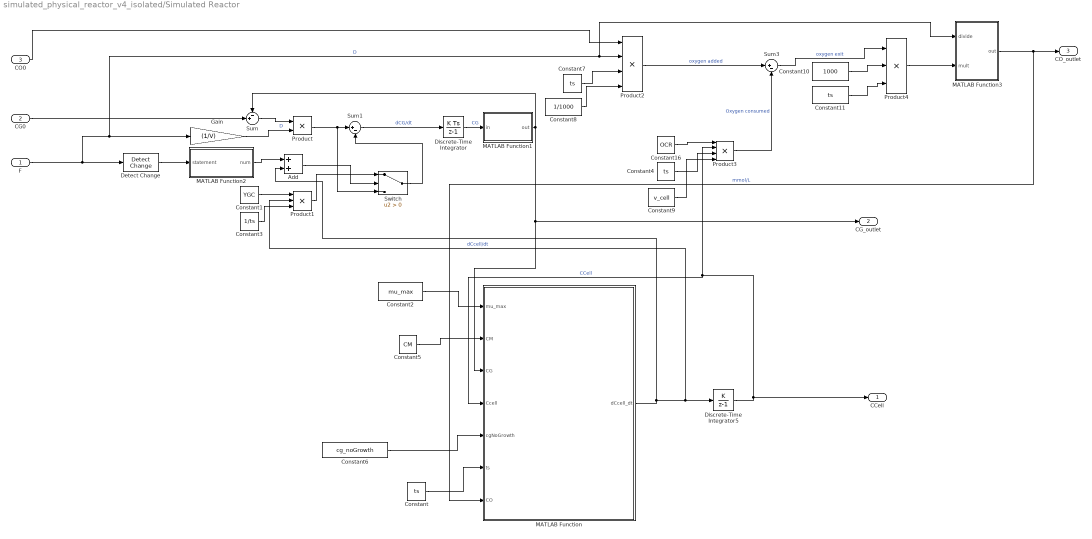
== system simulated_physical_reactor_v4_isolated/Simulated Reactor ==
  F : Inport
  CG0 : Inport  Port=2
  CO0 : Inport  Port=3
  Add : Sum
  Constant{,4,7,11} (4 alike) : Constant  Value=ts
  Constant1 : Constant  Value=YGC
  Constant10 : Constant  Value=1000
  Constant16 : Constant  Value=OCR
  Constant2 : Constant  Value=mu_max
  Constant3 : Constant  Value=1/ts
  Constant5 : Constant  Value=CM
  Constant6 : Constant  Value=cg_noGrowth
  Constant8 : Constant  Value=1/1000
  Constant9 : Constant  Value=v_cell
  Detect Change : simulink/Logic and Bit Operations/Detect Change  vinit=0  OutDataTypeStr=boolean
  Discrete-Time Integrator : DiscreteIntegrator  InitialCondition=CG0  SampleTime=ts  ICPrevOutput=DiscIntNeverNeededParam  ICPrevScaledInput=DiscIntNeverNeededParam
  Discrete-Time Integrator5 : DiscreteIntegrator  IntegratorMethod=Accumulation: Forward Euler  InitialCondition=Ccell0  SampleTime=ts  ICPrevOutput=DiscIntNeverNeededParam  ICPrevScaledInput=DiscIntNeverNeededParam
  Gain : Gain  Gain=(1/V)
  MATLAB Function : MATLAB Function  TreatAsAtomicUnit=on
  MATLAB Function1 : MATLAB Function  TreatAsAtomicUnit=on
  MATLAB Function2 : MATLAB Function  TreatAsAtomicUnit=on
  MATLAB Function3 : MATLAB Function  TreatAsAtomicUnit=on
  Product : Product
  Product1 : Product  Inputs=3
  Product2 : Product  Inputs=4
  Product3 : Product  Inputs=4
  Product4 : Product  Inputs=3
  Sum : Sum  Inputs=-+|
  Sum1 : Sum  Inputs=|+-
  Sum3 : Sum  Inputs=|+-
  Switch : Switch  Criteria=u2 > Threshold  SaturateOnIntegerOverflow=off  InputSameDT=off
  CCell : Outport
  CG_outlet : Outport  Port=2
  CO_outlet : Outport  Port=3
  wires:
  Discrete-Time Integrator5/1 -> Product3/2, MATLAB Function/4(Ccell), CCell/1  "CCell"
  MATLAB Function/1(dCcell_dt) -> Add/2, Product1/2, Discrete-Time Integrator5/1  "dCcell/dt"
  CG0/1 -> Sum/2
  Constant1/1 -> Product1/1
  Gain/1 -> Product/2  "D"
  Constant5/1 -> MATLAB Function/2(CM)
  Discrete-Time Integrator/1 -> MATLAB Function1/1(in)  "CG"
  Sum/1 -> Product/1
  Product/1 -> Switch/3, Sum1/1
  Constant2/1 -> MATLAB Function/1(mu_max)
  Product2/1 -> Sum3/1  "oxygen added"
  Constant16/1 -> Product3/1
  F/1 -> MATLAB Function3/1(divide), Product2/2, Gain/1, Detect Change/1  "D"
  Sum3/1 -> Product4/1  "oxygen exit"
  Sum1/1 -> Discrete-Time Integrator/1  "dCG/dt"
  Product1/1 -> Switch/1
  Detect Change/1 -> MATLAB Function2/1(statement)
  MATLAB Function2/1(num) -> Add/1
  Add/1 -> Switch/2
  CO0/1 -> Product2/1
  Product3/1 -> Sum3/2  "Oxygen consumed"
  Switch/1 -> Sum1/2
  Constant/1 -> MATLAB Function/6(ts)
  Constant3/1 -> Product1/3
  Constant4/1 -> Product3/3
  Constant6/1 -> MATLAB Function/5(cgNoGrowth)
  Constant7/1 -> Product2/3
  Constant8/1 -> Product2/4
  Constant9/1 -> Product3/4
  Product4/1 -> MATLAB Function3/2(mult)
  Constant10/1 -> Product4/2
  Constant11/1 -> Product4/3
  MATLAB Function3/1(out) -> MATLAB Function/7(CO), CO_outlet/1  "mmol/L"
  MATLAB Function1/1(out) -> Sum/1, MATLAB Function/3(CG), CG_outlet/1

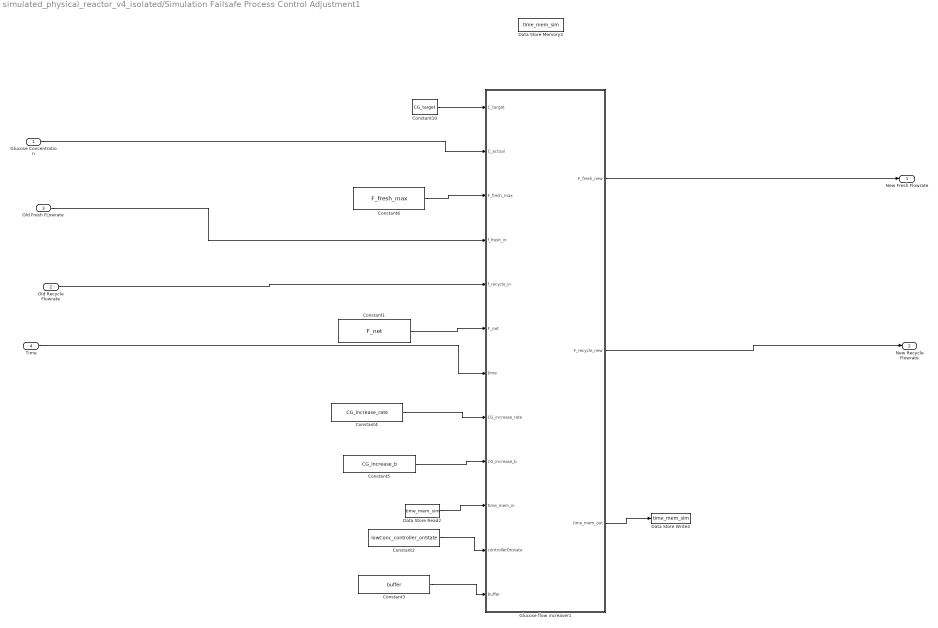
== system simulated_physical_reactor_v4_isolated/Simulation Failsafe Process Control Adjustment1 ==
  Glucose Concentration : Inport
  Old Recycle Flowrate : Inport  Port=2
  Old Fresh FLowrate : Inport  Port=3
  Time : Inport  Port=4
  Constant1 : Constant  Value=F_net
  Constant10 : Constant  Value=CG_target
  Constant2 : Constant  Value=lowConc_controller_onState
  Constant3 : Constant  Value=buffer
  Constant4 : Constant  Value=CG_increase_rate
  Constant5 : Constant  Value=CG_increase_b
  Constant6 : Constant  Value=F_fresh_max
  Data Store Memory2 : DataStoreMemory  DataStoreName=time_mem_sim  WriteAfterWriteMsg=warning  ShowAdditionalParam=off
  Data Store Read2 : DataStoreRead  DataStoreName=time_mem_sim  IndexOptions=Index vector (dialog)  Indices=1  OutputSizes=1
  Data Store Write2 : DataStoreWrite  DataStoreName=time_mem_sim  IndexOptions=Index vector (dialog)  Indices=1  OutputSizes=1
  Glucose flow increaser1 : MATLAB Function  TreatAsAtomicUnit=on
  New Fresh Flowrate : Outport
  New Recycle Flowrate : Outport  Port=2
  wires:
  Constant6/1 -> Glucose flow increaser1/3(F_fresh_max)
  Old Recycle Flowrate/1 -> Glucose flow increaser1/5(f_recycle_in)
  Old Fresh FLowrate/1 -> Glucose flow increaser1/4(f_fresh_in)
  Glucose flow increaser1/2(F_recycle_new) -> New Recycle Flowrate/1
  Constant2/1 -> Glucose flow increaser1/11(controllerOnstate)
  Constant5/1 -> Glucose flow increaser1/9(CG_increase_b)
  Data Store Read2/1 -> Glucose flow increaser1/10(time_mem_in)
  Constant4/1 -> Glucose flow increaser1/8(CG_increase_rate)
  Constant10/1 -> Glucose flow increaser1/1(C_target)
  Glucose Concentration/1 -> Glucose flow increaser1/2(C_actual)
  Constant1/1 -> Glucose flow increaser1/6(F_net)
  Glucose flow increaser1/3(time_mem_out) -> Data Store Write2/1
  Glucose flow increaser1/1(F_fresh_new) -> New Fresh Flowrate/1
  Time/1 -> Glucose flow increaser1/7(time)
  Constant3/1 -> Glucose flow increaser1/12(buffer)

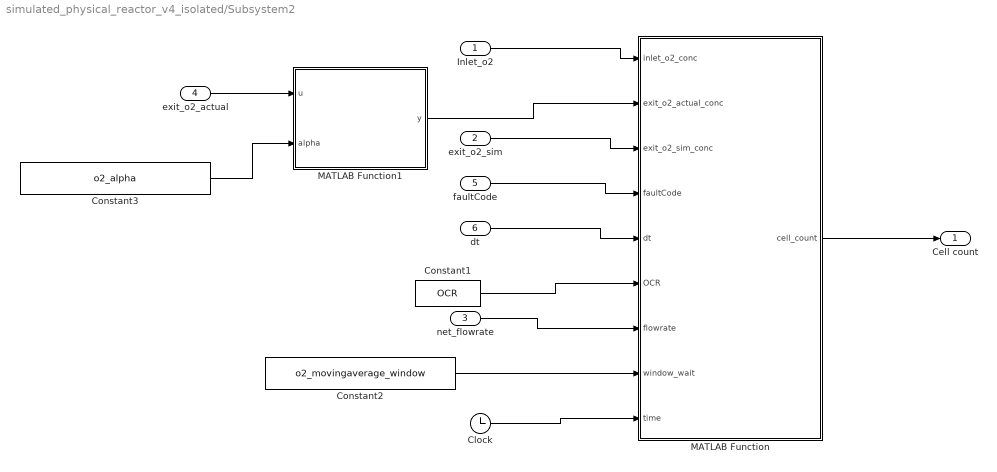
== system simulated_physical_reactor_v4_isolated/Subsystem2 ==
  Inlet_o2 : Inport
  exit_o2_sim : Inport  Port=2
  net_flowrate : Inport  Port=3
  exit_o2_actual : Inport  Port=4
  faultCode : Inport  Port=5
  dt : Inport  Port=6
  Clock : Clock
  Constant1 : Constant  Value=OCR
  Constant2 : Constant  Value=o2_movingaverage_window
  Constant3 : Constant  Value=o2_alpha
  MATLAB Function : MATLAB Function  TreatAsAtomicUnit=on
  MATLAB Function1 : MATLAB Function  TreatAsAtomicUnit=on
  Cell count : Outport
  wires:
  MATLAB Function/1(cell_count) -> Cell count/1
  Inlet_o2/1 -> MATLAB Function/1(inlet_o2_conc)
  exit_o2_sim/1 -> MATLAB Function/3(exit_o2_sim_conc)
  exit_o2_actual/1 -> MATLAB Function1/1(u)
  faultCode/1 -> MATLAB Function/4(faultCode)
  net_flowrate/1 -> MATLAB Function/7(flowrate)
  Constant1/1 -> MATLAB Function/6(OCR)
  dt/1 -> MATLAB Function/5(dt)
  Constant2/1 -> MATLAB Function/8(window_wait)
  Clock/1 -> MATLAB Function/9(time)
  MATLAB Function1/1(y) -> MATLAB Function/2(exit_o2_actual_conc)
  Constant3/1 -> MATLAB Function1/2(alpha)

== system simulated_physical_reactor_v4_isolated/Attack and Fault Detection System1/Fresh Pump Fault Detection ==
  fresh flowrate commanded : Inport
  glucose sensor concentration rolling average : Inport  Port=2
  dnr : Inport  Port=3
  Constant : Constant  Value=freshPump_response_window
  Constant1 : Constant  Value=freshPump_response_increases
  MATLAB Function : MATLAB Function  TreatAsAtomicUnit=on
  Moving Average : dspstat3/Moving Average  Method=Sliding window  ForgettingFactorPort=off  SpecifyWindowLength=on  WindowLength=g_flowrate_control_windowsize  OverlapLength=g_flowrate_control_windowsize-1  AllowArbitraryInputLength=off  ForgettingFactor=0.9  SimulateUsing=Code generation
  noFreshResponse : Outport
  wires:
  glucose sensor concentration rolling average/1 -> Moving Average/1
  fresh flowrate commanded/1 -> MATLAB Function/2(flowrate_commanded)
  Constant/1 -> MATLAB Function/4(samples_to_wait)
  Constant1/1 -> MATLAB Function/5(samples_increase_in_window)
  MATLAB Function/1(freshPumpFail) -> noFreshResponse/1
  Moving Average/1 -> MATLAB Function/3(glucose_sensor)
  dnr/1 -> MATLAB Function/1(dnr)
